simulink model "CSTR_sim"  (R2022b)
settings: Solver=ode8  StartTime=0.0  StopTime=t_end  FixedStep=Ts  RelTol=1e-3
undefined symbols (not defined in the file): A1, A2, A3, A4, A5, B1, B2, B3, B4, B5, C1, C2, C3, C4, C5, Ca, Cb, d1, D1, d2, D2, D3, D4, D5, Fa0, Fb0, K_sel, kv, kw, tFa_d_down, tFa_d_up, tFb_d_down, tFb_d_up, txa_r_down, txa_r_up, ty_r_down, ty_r_up, V, xa0, y0
settings Model: Creator=Ivona  LastModifiedBy=Milosh Yokich
settings SolverCC: AlgebraicLoopSolver=TrustRegion
settings DataIOCC: ReturnWorkspaceOutputs=off
settings DebuggingCC: UnconnectedInputMsg=warning  UnconnectedOutputMsg=warning  UnconnectedLineMsg=warning  SFMachineParentedDataDiag=warning  ArithmeticOperatorsInVariantConditions=warning
settings ModelReferenceCC: EnableRefExpFcnMdlSchedulingChecks=on
settings SFSimCC: SimUseLocalCustomCode=off  CustomCodeUndefinedFunction=UseInterfaceOnly
settings RTWCC: RTWUseLocalCustomCode=off
settings CodeAppCC: StateflowObjectComments=on
settings SimscapeCC: SimscapeNormalizeSystem=off

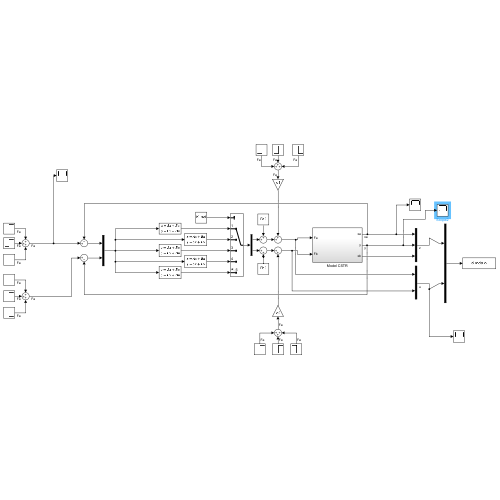
[thumbnail: Simulink's stored preview of the top-level diagram]
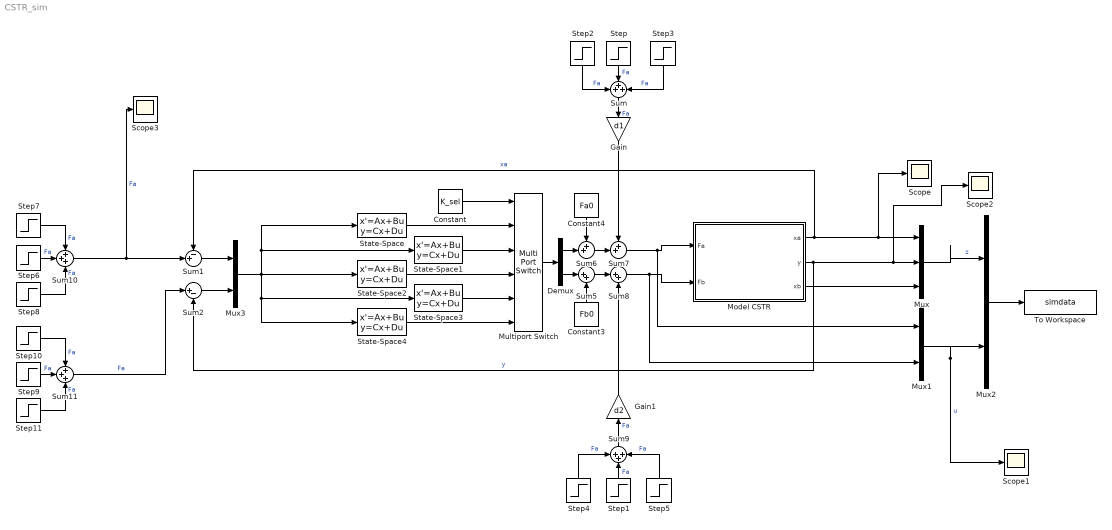
== system CSTR_sim ==
  Constant : Constant  Value=K_sel
  Constant3 : Constant  Value=Fb0
  Constant4 : Constant  Value=Fa0
  Demux : Demux  Outputs=2
  Gain : Gain  Gain=d1
  Gain1 : Gain  Gain=d2
  Model CSTR : Subsystem
  Multiport Switch : MultiPortSwitch  Inputs=5  SaturateOnIntegerOverflow=off  InputSameDT=off
  Mux : Mux  Inputs=3
  Mux1 : Mux  Inputs=2
  Mux2 : Mux  Inputs=2
  Mux3 : Mux  Inputs=2
  Scope{,1..3} (4 alike) : Scope
  State-Space : StateSpace  A=A1  B=B1  C=C1  D=D1  InitialCondition=0
  State-Space1 : StateSpace  A=A2  B=B2  C=C2  D=D2  InitialCondition=0
  State-Space2 : StateSpace  A=A3  B=B3  C=C3  D=D3  InitialCondition=0
  State-Space3 : StateSpace  A=A4  B=B4  C=C4  D=D4  InitialCondition=0
  State-Space4 : StateSpace  A=A5  B=B5  C=C5  D=D5  InitialCondition=0
  Step : Step  Time=0  After=0  SampleTime=0
  Step1 : Step  Time=0  After=0  SampleTime=0
  Step10 : Step  Time=ty_r_up  After=0.01*y0  SampleTime=0
  Step11 : Step  Time=ty_r_down  After=-0.01*y0  SampleTime=0
  Step2 : Step  Time=tFa_d_up  After=0.1*Fa0  SampleTime=0
  Step3 : Step  Time=tFa_d_down  After=-0.1*Fa0  SampleTime=0
  Step4 : Step  Time=tFb_d_up  After=0.1*Fb0  SampleTime=0
  Step5 : Step  Time=tFb_d_down  After=-0.1*Fb0  SampleTime=0
  Step6 : Step  Time=0  After=xa0  SampleTime=0
  Step7 : Step  Time=txa_r_up  After=0.1*xa0  SampleTime=0
  Step8 : Step  Time=txa_r_down  After=-0.1*xa0  SampleTime=0
  Step9 : Step  Time=0  After=y0  SampleTime=0
  Sum{,9..11} (4 alike) : Sum  Inputs=+++
  Sum1 : Sum  Inputs=-+|
  Sum2 : Sum  Inputs=|+-
  Sum5 : Sum  Inputs=|++
  Sum6 : Sum  Inputs=++|
  Sum7 : Sum  Inputs=++|
  Sum8 : Sum  Inputs=|++
  To Workspace : ToWorkspace  VariableName=simdata  SaveFormat=Timeseries  SampleTime=-1
  wires:
  Model CSTR/1(xa) -> Sum1/1, Mux/1, Scope/1  "xa"
  Model CSTR/2(y) -> Sum2/2, Mux/2, Scope2/1  "y"
  Mux/1 -> Mux2/1  "z"
  Mux1/1 -> Scope1/1, Mux2/2  "u"
  Mux2/1 -> To Workspace/1
  Step/1 -> Sum/2  "Fa"
  Step2/1 -> Sum/1  "Fa"
  Step3/1 -> Sum/3  "Fa"
  Model CSTR/3(xb) -> Mux/3
  Multiport Switch/1 -> Demux/1
  State-Space/1 -> Multiport Switch/2
  State-Space1/1 -> Multiport Switch/3
  State-Space2/1 -> Multiport Switch/4
  State-Space3/1 -> Multiport Switch/5
  State-Space4/1 -> Multiport Switch/6
  Constant/1 -> Multiport Switch/1
  Mux3/1 -> State-Space4/1, State-Space3/1, State-Space1/1, State-Space/1, State-Space2/1
  Sum1/1 -> Mux3/1
  Sum2/1 -> Mux3/2
  Demux/2 -> Sum5/1
  Demux/1 -> Sum6/2
  Constant3/1 -> Sum5/2
  Constant4/1 -> Sum6/1
  Sum6/1 -> Sum7/2
  Gain/1 -> Sum7/1
  Sum5/1 -> Sum8/1
  Sum7/1 -> Mux1/1, Model CSTR/1(Fa)
  Sum8/1 -> Mux1/2, Model CSTR/2(Fb)
  Gain1/1 -> Sum8/2
  Sum/1 -> Gain/1  "Fa"
  Step4/1 -> Sum9/1  "Fa"
  Step1/1 -> Sum9/2  "Fa"
  Step5/1 -> Sum9/3  "Fa"
  Sum9/1 -> Gain1/1  "Fa"
  Step7/1 -> Sum10/1  "Fa"
  Step6/1 -> Sum10/2  "Fa"
  Step8/1 -> Sum10/3  "Fa"
  Sum10/1 -> Scope3/1, Sum1/2  "Fa"
  Step10/1 -> Sum11/1  "Fa"
  Step9/1 -> Sum11/2  "Fa"
  Step11/1 -> Sum11/3  "Fa"
  Sum11/1 -> Sum2/1  "Fa"

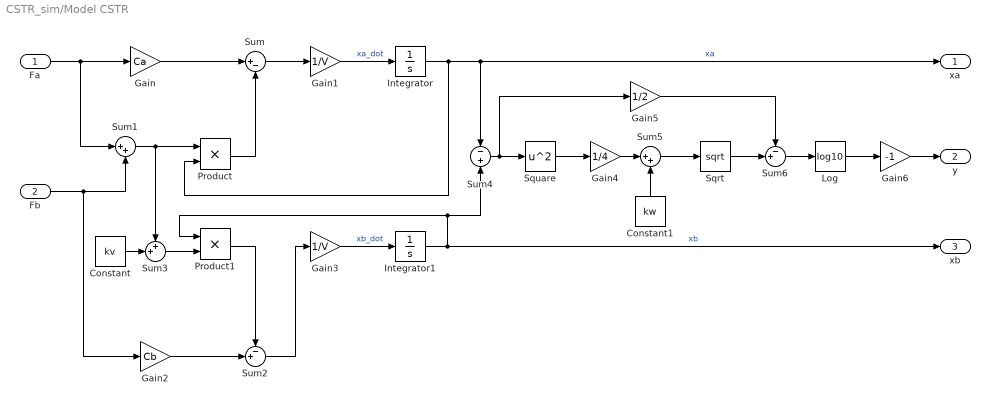
== system CSTR_sim/Model CSTR ==
  Fa : Inport
  Fb : Inport  Port=2
  Constant : Constant  Value=kv
  Constant1 : Constant  Value=kw
  Gain : Gain  Gain=Ca
  Gain1 : Gain  Gain=1/V
  Gain2 : Gain  Gain=Cb
  Gain3 : Gain  Gain=1/V
  Gain4 : Gain  Gain=1/4
  Gain5 : Gain  Gain=1/2
  Gain6 : Gain  Gain=-1
  Integrator : Integrator
  Integrator1 : Integrator
  Log : Math  Operator=log10  SignedPower=on
  Product : Product
  Product1 : Product
  Sqrt : Sqrt
  Square : Math  Operator=square  SignedPower=on
  Sum : Sum  Inputs=|+-
  Sum1 : Sum  Inputs=|++
  Sum2 : Sum  Inputs=-+|
  Sum3 : Sum  Inputs=++|
  Sum4 : Sum  Inputs=-+
  Sum5 : Sum  Inputs=|++
  Sum6 : Sum  Inputs=-+|
  xa : Outport
  y : Outport  Port=2
  xb : Outport  Port=3
  wires:
  Integrator/1 -> Product/2, Sum4/1, xa/1  "xa"
  Fa/1 -> Sum1/1, Gain/1
  Gain/1 -> Sum/1
  Fb/1 -> Gain2/1, Sum1/2
  Sum1/1 -> Sum3/1, Product/1
  Product/1 -> Sum/2
  Sum/1 -> Gain1/1
  Gain1/1 -> Integrator/1  "xa_dot"
  Gain2/1 -> Sum2/2
  Constant/1 -> Sum3/2
  Product1/1 -> Sum2/1
  Sum2/1 -> Gain3/1
  Integrator1/1 -> xb/1, Sum4/2, Product1/1  "xb"
  Sum3/1 -> Product1/2
  Gain3/1 -> Integrator1/1  "xb_dot"
  Square/1 -> Gain4/1
  Gain4/1 -> Sum5/1
  Constant1/1 -> Sum5/2
  Sum5/1 -> Sqrt/1
  Sqrt/1 -> Sum6/2
  Gain5/1 -> Sum6/1
  Sum6/1 -> Log/1
  Log/1 -> Gain6/1
  Gain6/1 -> y/1
  Sum4/1 -> Gain5/1, Square/1
